simulink model "quadcopterR2"  (R2022b)
settings: Solver=VariableStepAuto  StartTime=0.0  StopTime=10  RelTol=1e-3
values from neighbouring files (symbols this model uses):
  Az = sys_z.A    [quadcopter_analysis.m]
  Bz = sys_z.B    [quadcopter_analysis.m]
  Cz = sys_z.C    [quadcopter_analysis.m]
  Dz = sys_z.D    [quadcopter_analysis.m]
  phi_init = 0    [quadcopter_analysis.m]
  psi_init = 0    [quadcopter_analysis.m]
  theta_init = 0    [quadcopter_analysis.m]
  TS = 0.02    [quadcopter_analysis.m]
settings Model: Creator=collinlove  LastModifiedBy=E

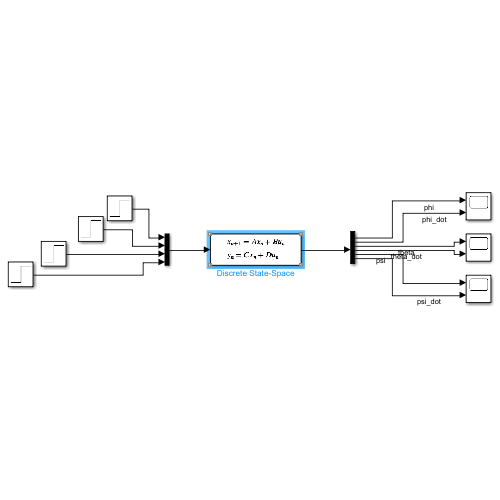
[thumbnail: Simulink's stored preview of the top-level diagram]
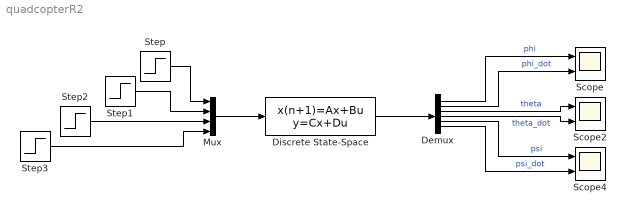
== system quadcopterR2 ==
  Demux : Demux  Outputs=6
  Discrete State-Space : DiscreteStateSpace  A=Az  B=Bz  C=Cz  D=Dz  InitialCondition=[phi_init,0,theta_init,0,psi_init,0]  SampleTime=TS
  Mux : Mux
  Scope : Scope  NumInputPorts=2
  Scope2 : Scope  NumInputPorts=2
  Scope4 : Scope  NumInputPorts=2
  Step{,1..3} (4 alike) : Step  Before=1  SampleTime=0
  wires:
  Mux/1 -> Discrete State-Space/1
  Step/1 -> Mux/1
  Step1/1 -> Mux/2
  Step2/1 -> Mux/3
  Step3/1 -> Mux/4
  Discrete State-Space/1 -> Demux/1
  Demux/1 -> Scope/1  "phi"
  Demux/2 -> Scope/2  "phi_dot"
  Demux/3 -> Scope2/1  "theta"
  Demux/4 -> Scope2/2  "theta_dot"
  Demux/5 -> Scope4/1  "psi"
  Demux/6 -> Scope4/2  "psi_dot"
